simulink library "MaskRadioButtons_library"  (R2018b)
settings: Solver=VariableStepAuto  StartTime=0.0  StopTime=10.0  RelTol=1e-3
settings Model: Creator=Christopher  LastModifiedBy=Christopher

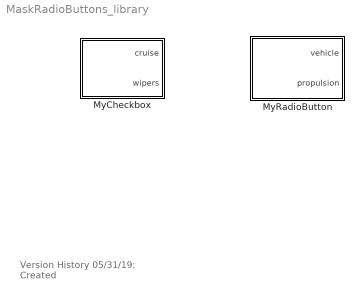
== system MaskRadioButtons_library ==
  note: Version History
      | 05/31/19: Created
  MyCheckbox : Subsystem  mask{cruiseControl=on, windshieldWipers=on}
      mask prompts: cruiseControl "Cruise control active?"; windshieldWipers "Windshield wipers active?"
      mask help: Illustrate how to use a 'Check Box' parameter.
  MyRadioButton : Subsystem  mask{vehicle=Aircraft, engineSystem=Gas}
      mask prompts: vehicle "Vehicle Type"; engineSystem "Engine System"
      mask help: Illustrate how to use the 'Radio Button' in a masked subsystem.
      mask TypeOptions vehicle: Aircraft | Boat | Car
      mask TypeOptions engineSystem: Gas | Electric | Hybrid | Squirrel

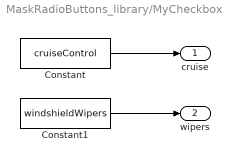
== system MaskRadioButtons_library/MyCheckbox ==
  Constant : Constant  Value=cruiseControl
  Constant1 : Constant  Value=windshieldWipers
  cruise : Outport
  wipers : Outport  Port=2
  wires:
  Constant/1 -> cruise/1
  Constant1/1 -> wipers/1

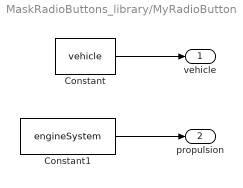
== system MaskRadioButtons_library/MyRadioButton ==
  Constant : Constant  Value=vehicle
  Constant1 : Constant  Value=engineSystem
  vehicle : Outport
  propulsion : Outport  Port=2
  wires:
  Constant/1 -> vehicle/1
  Constant1/1 -> propulsion/1
